simulink model "room_temp"  (R2024b)
settings: Solver=VariableStepAuto  StartTime=0.0  StopTime=10  RelTol=1e-3
settings Model: Creator=user  LastModifiedBy=user

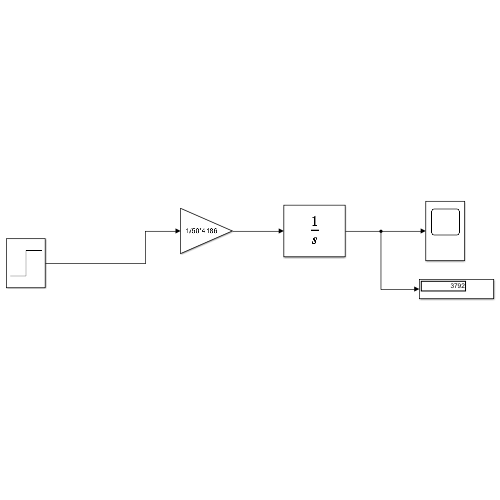
[thumbnail: Simulink's stored preview of the top-level diagram]
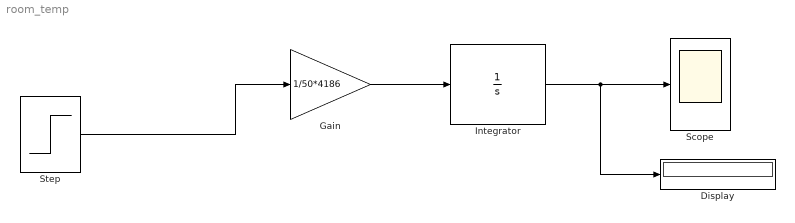
== system room_temp ==
  Display : Display
  Gain : Gain  Gain=1/50*4186
  Integrator : Integrator  InitialCondition=25
  Scope : Scope
  Step : Step  After=5  SampleTime=0
  wires:
  Gain/1 -> Integrator/1
  Integrator/1 -> Display/1, Scope/1
  Step/1 -> Gain/1
